simulink subsystem "Day1_Scenario_2"  (R2024a)
settings: Solver=VariableStepAuto  StartTime=0.0  StopTime=10.0  RelTol=1e-3
libraries: CarMaker4SL x2
settings Model: Creator=junhyung.cha  LastModifiedBy=User

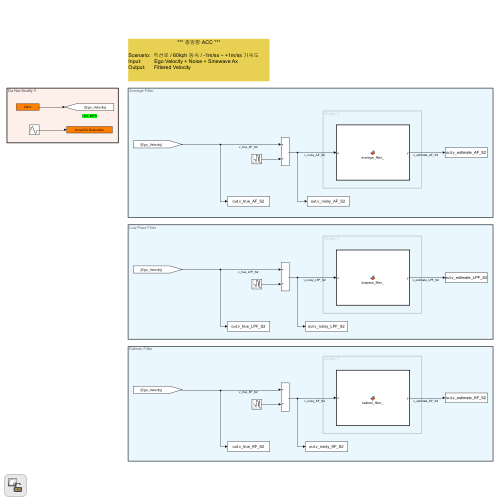
[thumbnail: Simulink's stored preview of the top-level diagram]
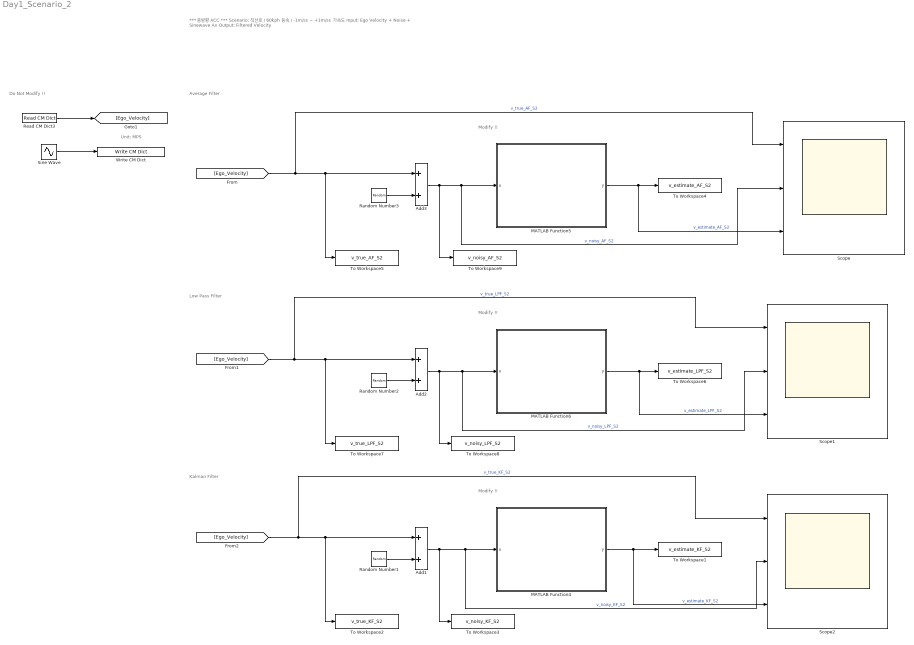
== system Day1_Scenario_2 ==
  note: Do Not Modify !!
  note: Low Pass Filter
  note: Average Filter
  note: Modify !!
  note: Modify !!
  note: Kalman Filter
  note: Modify !!
  note: *** 종방향 ACC ***
      |
      | Scenario: 직선로 / 60kph 등속 / -1m/ss ~ +1m/ss 가속도
      | Input: Ego Velocity + Noise + Sinewave Ax
      | Output: Filtered Velocity
  note: Unit: MPS
  Add1 : Sum
  Add2 : Sum
  Add3 : Sum
  MATLAB Function4 : MATLAB Function  TreatAsAtomicUnit=on
  MATLAB Function5 : MATLAB Function  TreatAsAtomicUnit=on
  MATLAB Function6 : MATLAB Function  TreatAsAtomicUnit=on
  Random Number1 : RandomNumber
  Random Number2 : RandomNumber
  Random Number3 : RandomNumber
  Read CM Dict3 : CarMaker4SL/Read CM Dict  xname=Car.v  xsync=off  xstime=Inherited
  Scope : Scope  NumInputPorts=3
  Scope1 : Scope  NumInputPorts=3
  Scope2 : Scope  NumInputPorts=3
  Sine Wave : Sin
  To Workspace1 : ToWorkspace  VariableName=v_estimate_KF_S2  SaveFormat=Timeseries  SampleTime=-1
  To Workspace2 : ToWorkspace  VariableName=v_true_KF_S2  SaveFormat=Timeseries  SampleTime=-1
  To Workspace3 : ToWorkspace  VariableName=v_noisy_KF_S2  SaveFormat=Timeseries  SampleTime=-1
  To Workspace4 : ToWorkspace  VariableName=v_estimate_AF_S2  SaveFormat=Timeseries  SampleTime=-1
  To Workspace5 : ToWorkspace  VariableName=v_true_AF_S2  SaveFormat=Timeseries  SampleTime=-1
  To Workspace6 : ToWorkspace  VariableName=v_estimate_LPF_S2  SaveFormat=Timeseries  SampleTime=-1
  To Workspace7 : ToWorkspace  VariableName=v_true_LPF_S2  SaveFormat=Timeseries  SampleTime=-1
  To Workspace8 : ToWorkspace  VariableName=v_noisy_LPF_S2  SaveFormat=Timeseries  SampleTime=-1
  To Workspace9 : ToWorkspace  VariableName=v_noisy_AF_S2  SaveFormat=Timeseries  SampleTime=-1
  Write CM Dict : CarMaker4SL/Write CM Dict  xname=AccelCtrl.DesiredAx  xsync=off
  wires:
  Sine Wave/1 -> Write CM Dict/1
  Random Number3/1 -> Add3/2
  Add3/1 -> To Workspace9/1, MATLAB Function5/1(u), Scope/2  "v_noisy_AF_S2"
  Add2/1 -> To Workspace8/1, MATLAB Function6/1(u), Scope1/2  "v_noisy_LPF_S2"
  [Ego_Velocity] -> Add2/1, To Workspace7/1, Scope1/1  "v_true_LPF_S2"
  MATLAB Function6/1(y) -> To Workspace6/1, Scope1/3  "v_estimate_LPF_S2"
  Random Number2/1 -> Add2/2
  MATLAB Function5/1(y) -> To Workspace4/1, Scope/3  "v_estimate_AF_S2"
  Add1/1 -> To Workspace3/1, MATLAB Function4/1(u), Scope2/2  "v_noisy_KF_S2"
  [Ego_Velocity] -> Add1/1, To Workspace2/1, Scope2/1  "v_true_KF_S2"
  MATLAB Function4/1(y) -> To Workspace1/1, Scope2/3  "v_estimate_KF_S2"
  [Ego_Velocity] -> Add3/1, To Workspace5/1, Scope/1  "v_true_AF_S2"
  Random Number1/1 -> Add1/2
  Read CM Dict3/1 -> [Ego_Velocity]

== matlab function Day1_Scenario_2/MATLAB Function5 ==
  settings: updateMethod=DISCRETE  sampleTime=0.05
  data: u input; y output
function y = exponential_moving_average(u)
    % 이동평균 필터 (실제로는 simple moving average임)
    persistent window num_average
    
    if isempty(window)
        num_average = 16;  % 원하면 기본값 변경 가능
        window = u;
    end
    
    window(end+1) = u;
    
    if length(window) > num_average
        window(1) = [];  % 가장 오래된 값 제거
    end
    
    y = mean(window);
end

== matlab function Day1_Scenario_2/MATLAB Function6 ==
  settings: updateMethod=DISCRETE  sampleTime=0.05
  data: u input; y output
function y = lowpass_filter_(u)
    persistent y_estimate alpha
    
    if isempty(y_estimate)
        alpha = 0.9;       % smoothing factor 초기값
        y_estimate = u;     % 첫 측정값 저장
    end
    
    y_estimate = alpha * y_estimate + (1 - alpha) * u;
    y = y_estimate;
end

== matlab function Day1_Scenario_2/MATLAB Function4 ==
  settings: updateMethod=DISCRETE  sampleTime=0.05
  data: u input; y output
function y = kalman_filter_(u)
    persistent A B C D Q R x_estimate P_estimate input_u
    
    if isempty(x_estimate)
        step_time = 0.1;
        m = 0.1;
        modelVariance = 0.01;
        measureVariance = 1.0;
        errorVariance_init = 10.0;
        
        A = 1.0;
        B = step_time / m;
        C = 1.0;
        D = 0.0;
        Q = modelVariance;
        R = measureVariance;
        
        x_estimate = u;
        P_estimate = errorVariance_init;
        
        input_u = 0;   % <<== input_u를 내부에서 상수로 지정
    end
    
    % Prediction
    x_pred = A * x_estimate + B * input_u;
    P_pred = A * P_estimate * A + Q;
    
    % Kalman Gain
    K = P_pred * C / (C * P_pred * C + R);
    
    % Update
    x_estimate = x_pred + K * (u - C * x_pred);
    P_estimate = (1 - K * C) * P_pred;
    
    y = x_estimate;
end
